simulink model "systemFixedSail"  (R2014b)
settings: Solver=ode3  StartTime=0.0  StopTime=10.0  FixedStep=0.1  RelTol=1e-3
settings Model: BufferReuse=off  Creator=paul  LastModifiedBy=Matthieu
settings DataIOCC: InitialState=[]  LoadInitialState=on  SaveOutput=off  SaveTime=off
settings OptimizationCC: InlineParams=on  BufferReuse=off
settings DebuggingCC: InitInArrayFormatMsg=none
settings RTWCC: GenerateReport=on  LaunchReport=on
settings GRTTargetCC: MatFileLogging=off

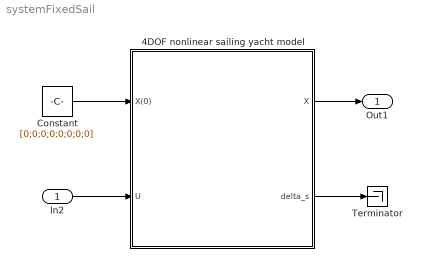
== system systemFixedSail ==
  In2 : Inport  PortDimensions=4
  4DOF nonlinear sailing yacht model : Subsystem
  Constant : Constant  Value=[0;0;0;0;0;0;0;0]
  Terminator : Terminator
  Out1 : Outport  PortDimensions=8
  wires:
  Constant/1 -> 4DOF nonlinear sailing yacht model/1(X(0))
  In2/1 -> 4DOF nonlinear sailing yacht model/2(U)
  4DOF nonlinear sailing yacht model/1(X) -> Out1/1
  4DOF nonlinear sailing yacht model/2(delta_s) -> Terminator/1

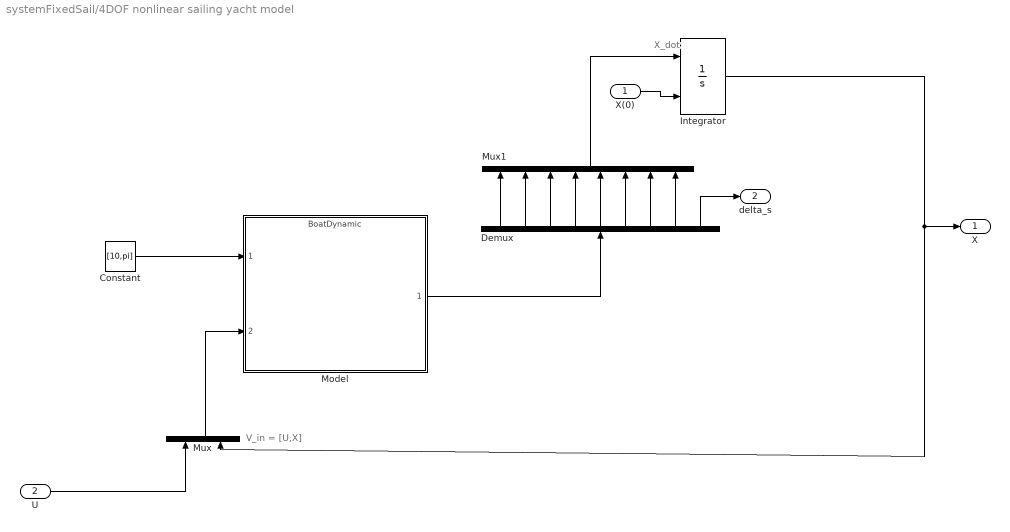
== system systemFixedSail/4DOF nonlinear sailing yacht model ==
  note: X_dot
  note: V_in = [U,X]
  X(0) : Inport
  U : Inport  Port=2
  Constant : Constant  Value=[10,pi]
  Demux : Demux  Outputs=9
  Integrator : Integrator  InitialConditionSource=external  InitialCondition=[0;0;0;pi;1;0;0;0]
  Model : ModelReference  ModelNameDialog=BoatDynamic.slx  SimulationMode=Normal  ModelReferenceVersion=1.9  CopyOfModelName=BoatDynamic.slx  DefaultDataLogging=on
  Mux : Mux  Inputs=2
  Mux1 : Mux  Inputs=8
  X : Outport
  delta_s : Outport  Port=2
  wires:
  X(0)/1 -> Integrator/2
  U/1 -> Mux/1
  Integrator/1 -> X/1, Mux/2
  Demux/9 -> delta_s/1
  Demux/8 -> Mux1/8
  Demux/7 -> Mux1/7
  Demux/6 -> Mux1/6
  Demux/5 -> Mux1/5
  Demux/4 -> Mux1/4
  Demux/3 -> Mux1/3
  Demux/2 -> Mux1/2
  Demux/1 -> Mux1/1
  Mux1/1 -> Integrator/1
  Constant/1 -> Model/1
  Mux/1 -> Model/2
  Model/1 -> Demux/1
